simulink model "simpSimuRoboToGo"  (R2019b)
settings: Solver=ode45  StartTime=0.0  StopTime=100.0  RelTol=1e-3  EnableMultiTasking=on
libraries: roblocks x1, simulink x1
settings Model: Creator=pic  LastModifiedBy=mackst
settings SolverCC: ZeroCrossAlgorithm=Adaptive
settings DataIOCC: SaveFormat=Array  TimeSaveName=t  OutputSaveName=y
settings OptimizationCC: ExpressionDepthLimit=2147483647  LifeSpan=inf
settings DebuggingCC: UnderspecifiedInitializationDetection=Classic  MergeDetectMultiDrivingBlocksExec=none  SolverPrmCheckMsg=warning  AllowSymbolicDim=off  StateNameClashWarn=warning  SFUnexpectedBacktrackingDiag=warning  SFNoUnconditionalDefaultTransitionDiag=warning  SFExecutionAtInitializationDiag=none  ArithmeticOperatorsInVariantConditions=warning
settings HardwareCC: ProdBitPerPointer=32  ProdBitPerSizeT=32  ProdBitPerPtrDiffT=32  ProdLargestAtomicFloat=None  ProdIntDivRoundTo=Undefined  ProdEndianess=Unspecified  ProdWordSize=32  ProdHWDeviceType=32-bit Generic
settings ModelReferenceCC: PropagateSignalLabelsOutOfModel=off
settings SFSimCC: SimUseLocalCustomCode=off  CustomCodeUndefinedFunction=UseInterfaceOnly
settings RTWCC: RTWUseLocalCustomCode=off
settings CodeAppCC: StateflowObjectComments=on
settings GRTTargetCC: TargetLangStandard=C89/C90 (ANSI)  GeneratePreprocessorConditionals=Disable all  CombineOutputUpdateFcns=off  GRTInterface=on
settings ConfigComp: CovMetricSettings=dw  CovHtmlReporting=on  CovSaveCumulativeToWorkspaceVar=on  CovSaveSingleToWorkspaceVar=on  CovExternalEMLEnable=off

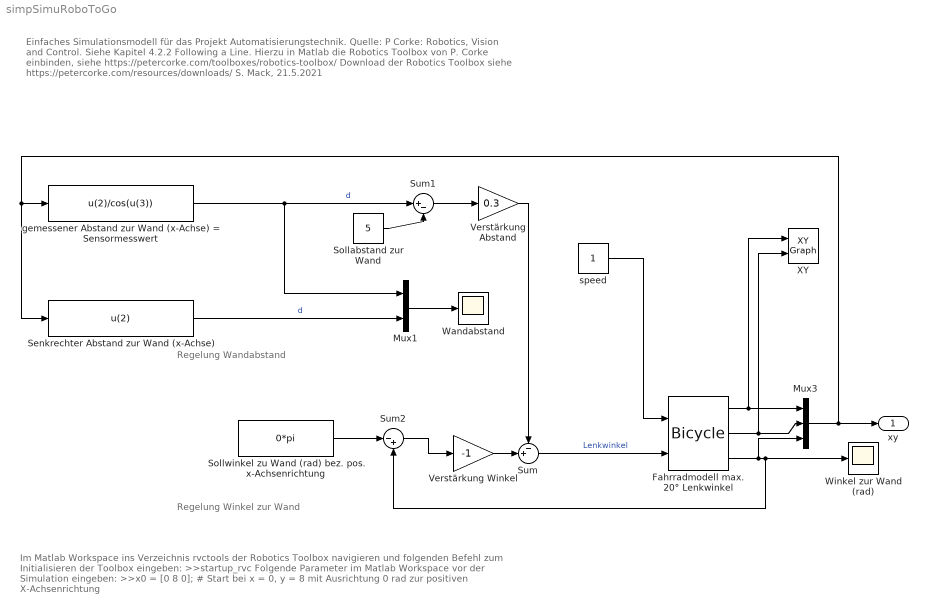
== system simpSimuRoboToGo ==
  note: Im Matlab Workspace ins Verzeichnis rvctools der Robotics Toolbox navigieren und folgenden Befehl zum Initialisieren der Toolbox eingeben:
      | >>startup_rvc
      | Folgende Parameter im Matlab Workspace vor der Simulation eingeben:
      | >>x0 = [0 8 0]; # Start bei x = 0, y = 8 mit Ausrichtung 0 rad zur positiven X-Achsenrichtung
  note: Regelung Wandabstand
  note: Regelung Winkel zur Wand
  note: Einfaches Simulationsmodell für das Projekt Automatisierungstechnik.
      | Quelle: P Corke: Robotics, Vision and Control. Siehe Kapitel 4.2.2 Following a Line.
      |
      | Hierzu in Matlab die Robotics Toolbox von P. Corke einbinden, siehe https://petercorke.com/toolboxes/robotics-toolbox/
      | Download der Robotics Toolbox siehe https://petercorke.com/resources/downloads/
      |
      | S. Mack, 21.5.2021
  Fahrradmodell max. 20° Lenkwinkel : roblocks/Vehicles/Bicycle  vlim=0.4  accel=1  alim=0.10  steer_rate=Inf  L=1  x0=x0
  Mux1 : Mux  Inputs=2
  Mux3 : Mux  Inputs=3
  Senkrechter Abstand zur Wand (x-Achse) : Fcn  Expr=u(2)
  Sollabstand zur Wand : Constant  Value=5
  Sollwinkel zu Wand (rad) bez. pos. x-Achsenrichtung : Constant  Value=0*pi
  Sum : Sum  Inputs=-+|
  Sum1 : Sum  Inputs=|+-
  Sum2 : Sum  Inputs=|-+
  Verstärkung Abstand : Gain  Gain=0.3
  Verstärkung Winkel : Gain  Gain=-1
  Wandabstand : Scope
  Winkel zur Wand (rad) : Scope
  XY : simulink/Sinks/XY Graph  xmin=0  xmax=40  ymin=0  ymax=10  st=-1
  gemessener Abstand zur Wand (x-Achse) = Sensormesswert : Fcn  Expr=u(2)/cos(u(3))
  speed : Constant  VectorParams1D=off  SampleTime=0.02
  xy : Outport  VectorParamsAs1DForOutWhenUnconnected=off
  wires:
  Mux3/1 -> Senkrechter Abstand zur Wand (x-Achse)/1, gemessener Abstand zur Wand (x-Achse) = Sensormesswert/1, xy/1
  Sollwinkel zu Wand (rad) bez. pos. x-Achsenrichtung/1 -> Sum2/1
  Verstärkung Winkel/1 -> Sum/2
  speed/1 -> Fahrradmodell max. 20° Lenkwinkel/1
  Sum/1 -> Fahrradmodell max. 20° Lenkwinkel/2  "Lenkwinkel"
  Fahrradmodell max. 20° Lenkwinkel/1 -> XY/1, Mux3/1
  Fahrradmodell max. 20° Lenkwinkel/2 -> XY/2, Mux3/2
  Fahrradmodell max. 20° Lenkwinkel/3 -> Sum2/2, Winkel zur Wand (rad)/1, Mux3/3
  Verstärkung Abstand/1 -> Sum/1
  Sum1/1 -> Verstärkung Abstand/1
  Sollabstand zur Wand/1 -> Sum1/2
  Mux1/1 -> Wandabstand/1
  gemessener Abstand zur Wand (x-Achse) = Sensormesswert/1 -> Mux1/1, Sum1/1  "d"
  Senkrechter Abstand zur Wand (x-Achse)/1 -> Mux1/2  "d"
  Sum2/1 -> Verstärkung Winkel/1
